simulink model "rc"  (Simulink 7.9)
settings: Solver=ode3  StartTime=0.0  StopTime=10.0  FixedStep=1e-5  RelTol=1e-3
undefined symbols (not defined in the file): c, r
settings Model: Creator=Daniel  LastModifiedBy=Daniel
settings DataIOCC: MaxDataPoints=1000000

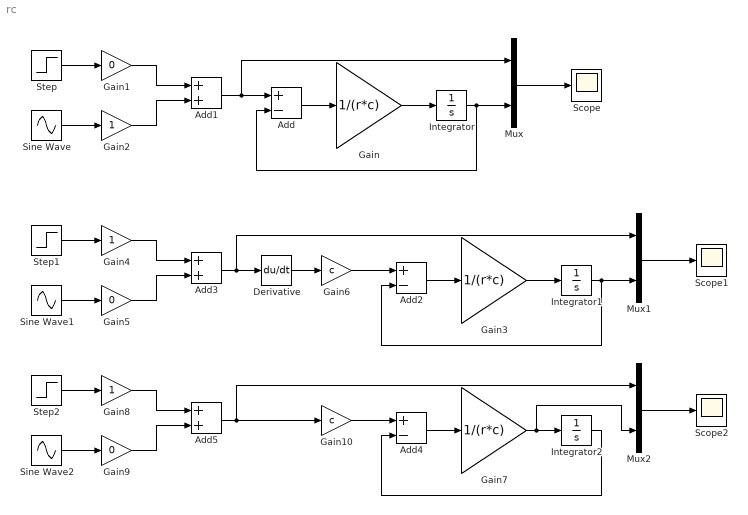
== system rc ==
  Add : Sum  Inputs=+-
  Add1 : Sum
  Add2 : Sum  Inputs=+-
  Add3 : Sum
  Add4 : Sum  Inputs=+-
  Add5 : Sum
  Derivative : Derivative
  Gain : Gain  Gain=1/(r*c)
  Gain1 : Gain  Gain=0
  Gain10 : Gain  Gain=c
  Gain2 : Gain
  Gain3 : Gain  Gain=1/(r*c)
  Gain4 : Gain
  Gain5 : Gain  Gain=0
  Gain6 : Gain  Gain=c
  Gain7 : Gain  Gain=1/(r*c)
  Gain8 : Gain
  Gain9 : Gain  Gain=0
  Integrator : Integrator
  Integrator1 : Integrator
  Integrator2 : Integrator
  Mux : Mux  Inputs=2
  Mux1 : Mux  Inputs=2
  Mux2 : Mux  Inputs=2
  Scope : Scope
  Scope1 : Scope
  Scope2 : Scope
      settings: SaveName=ScopeData2
  Sine Wave : Sin  Frequency=10  SampleTime=0
  Sine Wave1 : Sin  Frequency=10  SampleTime=0
  Sine Wave2 : Sin  Frequency=10  SampleTime=0
  Step : Step  SampleTime=0
  Step1 : Step  SampleTime=0
  Step2 : Step  SampleTime=0
  wires:
  Add/1 -> Gain/1
  Gain/1 -> Integrator/1
  Integrator/1 -> Add/2, Mux/2
  Mux/1 -> Scope/1
  Step/1 -> Gain1/1
  Sine Wave/1 -> Gain2/1
  Gain1/1 -> Add1/1
  Add1/1 -> Add/1, Mux/1
  Gain2/1 -> Add1/2
  Add2/1 -> Gain3/1
  Gain3/1 -> Integrator1/1
  Integrator1/1 -> Add2/2, Mux1/2
  Mux1/1 -> Scope1/1
  Step1/1 -> Gain4/1
  Sine Wave1/1 -> Gain5/1
  Gain4/1 -> Add3/1
  Add3/1 -> Derivative/1, Mux1/1
  Gain5/1 -> Add3/2
  Derivative/1 -> Gain6/1
  Gain6/1 -> Add2/1
  Add4/1 -> Gain7/1
  Integrator2/1 -> Add4/2
  Mux2/1 -> Scope2/1
  Step2/1 -> Gain8/1
  Sine Wave2/1 -> Gain9/1
  Gain8/1 -> Add5/1
  Add5/1 -> Mux2/1, Gain10/1
  Gain9/1 -> Add5/2
  Gain10/1 -> Add4/1
  Gain7/1 -> Integrator2/1, Mux2/2
